simulink model "test_final_sift"  (R2015a)
settings: Solver=ode45  StartTime=0.0  StopTime=10.0  RelTol=1e-3
InitFcn:
  | %% DSPBuilder Start
  | alt_dspbuilder_update_model(bdroot)
  | %% DSPBuilder End
libraries: allblocks_alteradspbuilder2 x2309
(part 2 of 27)

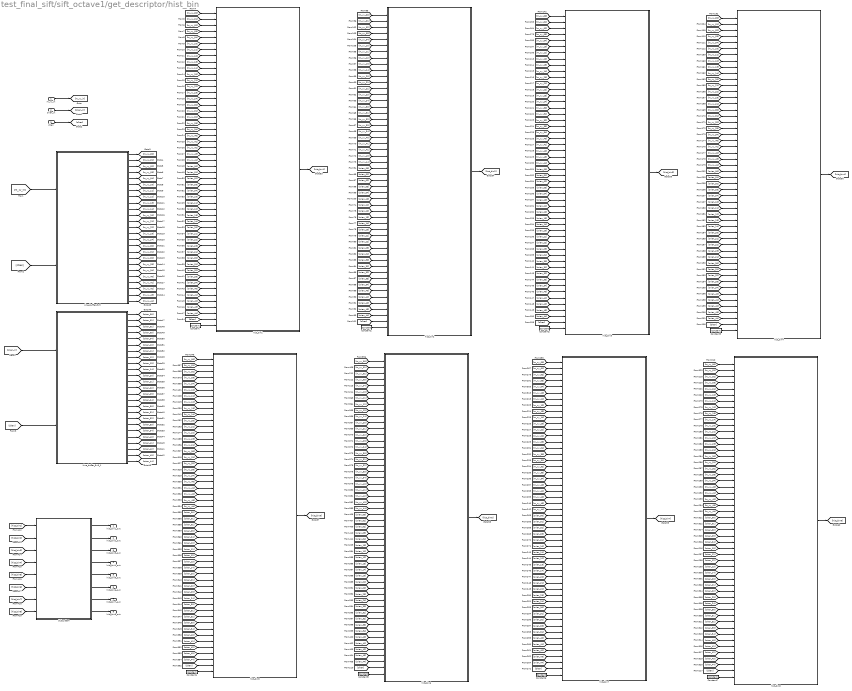
== system test_final_sift/sift_octave1/get_descriptor/hist_bin ==
  m_xy_In : Inport
  orien_In : Inport  Port=2
  clken : Inport  Port=3
  Constant : allblocks_alteradspbuilder2/Constant  mask_cst=1  BusType=Unsigned Integer  bwl=8  bwr=0  roundMode=Truncate  satMode=Wrap  SpecifyClock=off  allowFloatingPointOverride=on  logOutputs=off  logFile=C:\Users\ASUS\Desktop\sift_fpga\Octave_2\tb_test_final_sift\test%5Ffinal%5Fsift_sift%5Foctave1_get%5Fdescriptor_hist%5Fbin_Constant.fixedpointlog
  Constant1 : allblocks_alteradspbuilder2/Constant  mask_cst=2  BusType=Unsigned Integer  bwl=8  bwr=0  roundMode=Truncate  satMode=Wrap  SpecifyClock=off  allowFloatingPointOverride=on  logOutputs=off  logFile=C:\Users\ASUS\Desktop\sift_fpga\Octave_2\tb_test_final_sift\test%5Ffinal%5Fsift_sift%5Foctave1_get%5Fdescriptor_hist%5Fbin_Constant1.fixedpointlog
  Constant2 : allblocks_alteradspbuilder2/Constant  mask_cst=3  BusType=Unsigned Integer  bwl=8  bwr=0  roundMode=Truncate  satMode=Wrap  SpecifyClock=off  allowFloatingPointOverride=on  logOutputs=off  logFile=C:\Users\ASUS\Desktop\sift_fpga\Octave_2\tb_test_final_sift\test%5Ffinal%5Fsift_sift%5Foctave1_get%5Fdescriptor_hist%5Fbin_Constant2.fixedpointlog
  Constant3 : allblocks_alteradspbuilder2/Constant  mask_cst=4  BusType=Unsigned Integer  bwl=8  bwr=0  roundMode=Truncate  satMode=Wrap  SpecifyClock=off  allowFloatingPointOverride=on  logOutputs=off  logFile=C:\Users\ASUS\Desktop\sift_fpga\Octave_2\tb_test_final_sift\test%5Ffinal%5Fsift_sift%5Foctave1_get%5Fdescriptor_hist%5Fbin_Constant3.fixedpointlog
  Constant4 : allblocks_alteradspbuilder2/Constant  mask_cst=5  BusType=Unsigned Integer  bwl=8  bwr=0  roundMode=Truncate  satMode=Wrap  SpecifyClock=off  allowFloatingPointOverride=on  logOutputs=off  logFile=C:\Users\ASUS\Desktop\sift_fpga\Octave_2\tb_test_final_sift\test%5Ffinal%5Fsift_sift%5Foctave1_get%5Fdescriptor_hist%5Fbin_Constant4.fixedpointlog
  Constant5 : allblocks_alteradspbuilder2/Constant  mask_cst=6  BusType=Unsigned Integer  bwl=8  bwr=0  roundMode=Truncate  satMode=Wrap  SpecifyClock=off  allowFloatingPointOverride=on  logOutputs=off  logFile=C:\Users\ASUS\Desktop\sift_fpga\Octave_2\tb_test_final_sift\test%5Ffinal%5Fsift_sift%5Foctave1_get%5Fdescriptor_hist%5Fbin_Constant5.fixedpointlog
  Constant6 : allblocks_alteradspbuilder2/Constant  mask_cst=7  BusType=Unsigned Integer  bwl=8  bwr=0  roundMode=Truncate  satMode=Wrap  SpecifyClock=off  allowFloatingPointOverride=on  logOutputs=off  logFile=C:\Users\ASUS\Desktop\sift_fpga\Octave_2\tb_test_final_sift\test%5Ffinal%5Fsift_sift%5Foctave1_get%5Fdescriptor_hist%5Fbin_Constant6.fixedpointlog
  Constant7 : allblocks_alteradspbuilder2/Constant  mask_cst=8  BusType=Unsigned Integer  bwl=8  bwr=0  roundMode=Truncate  satMode=Wrap  SpecifyClock=off  allowFloatingPointOverride=on  logOutputs=off  logFile=C:\Users\ASUS\Desktop\sift_fpga\Octave_2\tb_test_final_sift\test%5Ffinal%5Fsift_sift%5Foctave1_get%5Fdescriptor_hist%5Fbin_Constant7.fixedpointlog
  Line_buffer_5x5 : Subsystem
  Line_buffer_5x5_1 : Subsystem
  Subsystem : Subsystem
  hist_bin1 : Subsystem
  hist_bin2 : Subsystem
  hist_bin3 : Subsystem
  hist_bin4 : Subsystem
  hist_bin5 : Subsystem
  hist_bin6 : Subsystem
  hist_bin7 : Subsystem
  hist_bin8 : Subsystem
  hist_bin1_out : Outport
  hist_bin2_out : Outport  Port=2
  hist_bin3_out : Outport  Port=3
  hist_bin4_out : Outport  Port=4
  hist_bin5_out : Outport  Port=5
  hist_bin6_out : Outport  Port=6
  hist_bin7_out : Outport  Port=7
  hist_bin8_out : Outport  Port=8
  wires:
  [hist_bin7] -> Subsystem/7(hist_in_bin7)
  [m_xy_in] -> Line_buffer_5x5/1(dataIn)
  [clken] -> Line_buffer_5x5/2(clken)
  [clken] -> Line_buffer_5x5_1/2(clken)
  [orien_in] -> Line_buffer_5x5_1/1(dataIn)
  clken/1 -> [clken]
  Line_buffer_5x5_1/21(Out40) -> [orien_40]
  Line_buffer_5x5_1/19(Out33) -> [orien_33]
  Line_buffer_5x5_1/8(Out12) -> [orien_12]
  Line_buffer_5x5_1/14(Out23) -> [orien_23]
  Line_buffer_5x5_1/18(Out32) -> [orien_32]
  Line_buffer_5x5_1/20(Out34) -> [orien_34]
  Line_buffer_5x5_1/2(Out01) -> [orien_01]
  Line_buffer_5x5_1/7(Out11) -> [orien_11]
  Line_buffer_5x5_1/11(Out20) -> [orien_20]
  Line_buffer_5x5_1/13(Out22) -> [orien_22]
  Line_buffer_5x5_1/17(Out31) -> [orien_31]
  Line_buffer_5x5_1/25(Out44) -> [orien_44]
  Line_buffer_5x5_1/3(Out02) -> [orien_02]
  Line_buffer_5x5_1/5(Out04) -> [orien_04]
  Line_buffer_5x5_1/23(Out42) -> [orien_42]
  Line_buffer_5x5_1/24(Out43) -> [orien_43]
  Line_buffer_5x5_1/6(Out10) -> [orien_10]
  Line_buffer_5x5_1/1(Out00) -> [orien_00]
  Line_buffer_5x5_1/22(Out41) -> [orien_41]
  Line_buffer_5x5_1/15(Out24) -> [orien_24]
  Line_buffer_5x5_1/4(Out03) -> [orien_03]
  Line_buffer_5x5_1/9(Out13) -> [orien_13]
  Line_buffer_5x5_1/10(Out14) -> [orien_14]
  Line_buffer_5x5_1/12(Out21) -> [orien_21]
  Line_buffer_5x5_1/16(Out30) -> [orien_30]
  Line_buffer_5x5/24(Out43) -> [m_xy_43]
  Line_buffer_5x5/21(Out40) -> [m_xy_40]
  Line_buffer_5x5/23(Out42) -> [m_xy_42]
  Line_buffer_5x5/22(Out41) -> [m_xy_41]
  Line_buffer_5x5/25(Out44) -> [m_xy_44]
  Line_buffer_5x5/12(Out21) -> [m_xy_21]
  Line_buffer_5x5/15(Out24) -> [m_xy_24]
  Line_buffer_5x5/19(Out33) -> [m_xy_33]
  Line_buffer_5x5/18(Out32) -> [m_xy_32]
  Line_buffer_5x5/13(Out22) -> [m_xy_22]
  Line_buffer_5x5/11(Out20) -> [m_xy_20]
  Line_buffer_5x5/16(Out30) -> [m_xy_30]
  Line_buffer_5x5/14(Out23) -> [m_xy_23]
  Line_buffer_5x5/17(Out31) -> [m_xy_31]
  Line_buffer_5x5/20(Out34) -> [m_xy_34]
  [hist_bin1] -> Subsystem/1(hist_in_bin1)
  Line_buffer_5x5/1(Out00) -> [m_xy_00]
  [m_xy_04] -> hist_bin1/5(Mxy_In04)
  Line_buffer_5x5/2(Out01) -> [m_xy_01]
  hist_bin1/1(bin_out) -> [hist_bin1]
  [m_xy_10] -> hist_bin1/6(Mxy_In10)
  Line_buffer_5x5/9(Out13) -> [m_xy_13]
  [m_xy_13] -> hist_bin1/9(Mxy_In13)
  Line_buffer_5x5/10(Out14) -> [m_xy_14]
  Line_buffer_5x5/6(Out10) -> [m_xy_10]
  Line_buffer_5x5/7(Out11) -> [m_xy_11]
  [m_xy_11] -> hist_bin1/7(Mxy_In11)
  [m_xy_12] -> hist_bin1/8(Mxy_In12)
  Line_buffer_5x5/8(Out12) -> [m_xy_12]
  [m_xy_14] -> hist_bin1/10(Mxy_In14)
  [m_xy_22] -> hist_bin1/13(Mxy_In22)
  [m_xy_40] -> hist_bin1/21(Mxy_In40)
  [m_xy_43] -> hist_bin1/24(Mxy_In43)
  [m_xy_42] -> hist_bin1/23(Mxy_In42)
  [m_xy_44] -> hist_bin1/25(Mxy_In44)
  [m_xy_24] -> hist_bin1/15(Mxy_In24)
  [m_xy_21] -> hist_bin1/12(Mxy_In21)
  [m_xy_20] -> hist_bin1/11(Mxy_In20)
  [m_xy_23] -> hist_bin1/14(Mxy_In23)
  [m_xy_41] -> hist_bin1/22(Mxy_In41)
  [m_xy_01] -> hist_bin1/2(Mxy_In01)
  Line_buffer_5x5/4(Out03) -> [m_xy_03]
  Line_buffer_5x5/5(Out04) -> [m_xy_04]
  Line_buffer_5x5/3(Out02) -> [m_xy_02]
  [m_xy_31] -> hist_bin1/17(Mxy_In31)
  [m_xy_30] -> hist_bin1/16(Mxy_In30)
  [m_xy_34] -> hist_bin1/20(Mxy_In34)
  [m_xy_33] -> hist_bin1/19(Mxy_In33)
  [m_xy_32] -> hist_bin1/18(Mxy_In32)
  [m_xy_03] -> hist_bin1/4(Mxy_In03)
  [m_xy_02] -> hist_bin1/3(Mxy_In02)
  [hist_bin3] -> Subsystem/3(hist_in_bin3)
  [hist_bin4] -> Subsystem/4(hist_in_bin4)
  [orien_10] -> hist_bin1/31(Orien_In10)
  [orien_42] -> hist_bin1/48(Orien_In42)
  [orien_01] -> hist_bin1/27(Orien_In01)
  [orien_20] -> hist_bin1/36(Orien_In20)
  [orien_31] -> hist_bin1/42(Orien_In31)
  [orien_33] -> hist_bin1/44(Orien_In33)
  [orien_21] -> hist_bin1/37(Orien_In21)
  [orien_24] -> hist_bin1/40(Orien_In24)
  [orien_03] -> hist_bin1/29(Orien_In03)
  [orien_30] -> hist_bin1/41(Orien_In30)
  [orien_12] -> hist_bin1/33(Orien_In12)
  [orien_23] -> hist_bin1/39(Orien_In23)
  [orien_32] -> hist_bin1/43(Orien_In32)
  [orien_41] -> hist_bin1/47(Orien_In41)
  [orien_43] -> hist_bin1/49(Orien_In43)
  [orien_02] -> hist_bin1/28(Orien_In02)
  [orien_00] -> hist_bin1/26(Orien_In00)
  [orien_11] -> hist_bin1/32(Orien_In11)
  [orien_34] -> hist_bin1/45(Orien_In34)
  [orien_22] -> hist_bin1/38(Orien_In22)
  [orien_04] -> hist_bin1/30(Orien_In04)
  [orien_14] -> hist_bin1/35(Orien_In14)
  [orien_44] -> hist_bin1/50(Orien_In44)
  [orien_13] -> hist_bin1/34(Orien_In13)
  [orien_40] -> hist_bin1/46(Orien_In40)
  [clken] -> hist_bin1/51(clken)
  Constant/1 -> hist_bin1/52(bin_in)
  [m_xy_02] -> hist_bin2/3(Mxy_In02)
  [m_xy_04] -> hist_bin2/5(Mxy_In04)
  [m_xy_10] -> hist_bin2/6(Mxy_In10)
  [m_xy_23] -> hist_bin2/14(Mxy_In23)
  [m_xy_31] -> hist_bin2/17(Mxy_In31)
  [m_xy_30] -> hist_bin2/16(Mxy_In30)
  [m_xy_12] -> hist_bin2/8(Mxy_In12)
  [m_xy_32] -> hist_bin2/18(Mxy_In32)
  [m_xy_13] -> hist_bin2/9(Mxy_In13)
  [m_xy_33] -> hist_bin2/19(Mxy_In33)
  [m_xy_41] -> hist_bin2/22(Mxy_In41)
  [m_xy_01] -> hist_bin2/2(Mxy_In01)
  [m_xy_14] -> hist_bin2/10(Mxy_In14)
  [m_xy_40] -> hist_bin2/21(Mxy_In40)
  [m_xy_43] -> hist_bin2/24(Mxy_In43)
  [m_xy_20] -> hist_bin2/11(Mxy_In20)
  [m_xy_22] -> hist_bin2/13(Mxy_In22)
  [m_xy_24] -> hist_bin2/15(Mxy_In24)
  [m_xy_34] -> hist_bin2/20(Mxy_In34)
  [m_xy_03] -> hist_bin2/4(Mxy_In03)
  [m_xy_00] -> hist_bin2/1(Mxy_In00)
  [m_xy_11] -> hist_bin2/7(Mxy_In11)
  [m_xy_21] -> hist_bin2/12(Mxy_In21)
  [orien_31] -> hist_bin2/42(Orien_In31)
  [orien_34] -> hist_bin2/45(Orien_In34)
  [m_xy_42] -> hist_bin2/23(Mxy_In42)
  [orien_01] -> hist_bin2/27(Orien_In01)
  [orien_00] -> hist_bin2/26(Orien_In00)
  [orien_04] -> hist_bin2/30(Orien_In04)
  [orien_13] -> hist_bin2/34(Orien_In13)
  [orien_20] -> hist_bin2/36(Orien_In20)
  [orien_24] -> hist_bin2/40(Orien_In24)
  [orien_33] -> hist_bin2/44(Orien_In33)
  [orien_32] -> hist_bin2/43(Orien_In32)
  [orien_41] -> hist_bin2/47(Orien_In41)
  [orien_11] -> hist_bin2/32(Orien_In11)
  [orien_21] -> hist_bin2/37(Orien_In21)
  [orien_14] -> hist_bin2/35(Orien_In14)
  [orien_22] -> hist_bin2/38(Orien_In22)
  [orien_23] -> hist_bin2/39(Orien_In23)
  [orien_02] -> hist_bin2/28(Orien_In02)
  [orien_10] -> hist_bin2/31(Orien_In10)
  [orien_12] -> hist_bin2/33(Orien_In12)
  [orien_30] -> hist_bin2/41(Orien_In30)
  [m_xy_44] -> hist_bin2/25(Mxy_In44)
  [orien_03] -> hist_bin2/29(Orien_In03)
  [orien_40] -> hist_bin2/46(Orien_In40)
  [clken] -> hist_bin2/51(clken)
  hist_bin2/1(bin_out) -> [hist_bin2]
  [orien_42] -> hist_bin2/48(Orien_In42)
  [orien_44] -> hist_bin2/50(Orien_In44)
  [orien_43] -> hist_bin2/49(Orien_In43)
  Constant1/1 -> hist_bin2/52(bin_in)
  [m_xy_00] -> hist_bin1/1(Mxy_In00)
  Subsystem/4(bin4_out) -> hist_bin4_out/1
  Subsystem/3(bin3_out) -> hist_bin3_out/1
  [hist_bin8] -> Subsystem/8(hist_in_bin8)
  [hist_bin6] -> Subsystem/6(hist_in_bin6)
  [hist_bin5] -> Subsystem/5(hist_in_bin5)
  Subsystem/2(bin2_out) -> hist_bin2_out/1
  orien_In/1 -> [orien_in]
  m_xy_In/1 -> [m_xy_in]
  Subsystem/5(bin5_out) -> hist_bin5_out/1
  Subsystem/6(bin6_out) -> hist_bin6_out/1
  Subsystem/7(bin7_out) -> hist_bin7_out/1
  Subsystem/8(bin8_out) -> hist_bin8_out/1
  [hist_bin2] -> Subsystem/2(hist_in_bin2)
  [m_xy_04] -> hist_bin3/5(Mxy_In04)
  hist_bin3/1(bin_out) -> [hist_bin3]
  [m_xy_10] -> hist_bin3/6(Mxy_In10)
  [m_xy_13] -> hist_bin3/9(Mxy_In13)
  [m_xy_11] -> hist_bin3/7(Mxy_In11)
  [m_xy_12] -> hist_bin3/8(Mxy_In12)
  [m_xy_14] -> hist_bin3/10(Mxy_In14)
  [m_xy_22] -> hist_bin3/13(Mxy_In22)
  [m_xy_40] -> hist_bin3/21(Mxy_In40)
  [m_xy_43] -> hist_bin3/24(Mxy_In43)
  [m_xy_42] -> hist_bin3/23(Mxy_In42)
  [m_xy_44] -> hist_bin3/25(Mxy_In44)
  [m_xy_24] -> hist_bin3/15(Mxy_In24)
  [m_xy_21] -> hist_bin3/12(Mxy_In21)
  [m_xy_20] -> hist_bin3/11(Mxy_In20)
  [m_xy_23] -> hist_bin3/14(Mxy_In23)
  [m_xy_41] -> hist_bin3/22(Mxy_In41)
  [m_xy_01] -> hist_bin3/2(Mxy_In01)
  [m_xy_31] -> hist_bin3/17(Mxy_In31)
  [m_xy_30] -> hist_bin3/16(Mxy_In30)
  [m_xy_34] -> hist_bin3/20(Mxy_In34)
  [m_xy_33] -> hist_bin3/19(Mxy_In33)
  [m_xy_32] -> hist_bin3/18(Mxy_In32)
  [m_xy_03] -> hist_bin3/4(Mxy_In03)
  [m_xy_02] -> hist_bin3/3(Mxy_In02)
  [orien_10] -> hist_bin3/31(Orien_In10)
  [orien_42] -> hist_bin3/48(Orien_In42)
  [orien_01] -> hist_bin3/27(Orien_In01)
  [orien_20] -> hist_bin3/36(Orien_In20)
  [orien_31] -> hist_bin3/42(Orien_In31)
  [orien_33] -> hist_bin3/44(Orien_In33)
  [orien_21] -> hist_bin3/37(Orien_In21)
  [orien_24] -> hist_bin3/40(Orien_In24)
  [orien_03] -> hist_bin3/29(Orien_In03)
  [orien_30] -> hist_bin3/41(Orien_In30)
  [orien_12] -> hist_bin3/33(Orien_In12)
  [orien_23] -> hist_bin3/39(Orien_In23)
  [orien_32] -> hist_bin3/43(Orien_In32)
  [orien_41] -> hist_bin3/47(Orien_In41)
  [orien_43] -> hist_bin3/49(Orien_In43)
  [orien_02] -> hist_bin3/28(Orien_In02)
  [orien_00] -> hist_bin3/26(Orien_In00)
  [orien_11] -> hist_bin3/32(Orien_In11)
  [orien_34] -> hist_bin3/45(Orien_In34)
  [orien_22] -> hist_bin3/38(Orien_In22)
  [orien_04] -> hist_bin3/30(Orien_In04)
  [orien_14] -> hist_bin3/35(Orien_In14)
  [orien_44] -> hist_bin3/50(Orien_In44)
  [orien_13] -> hist_bin3/34(Orien_In13)
  [orien_40] -> hist_bin3/46(Orien_In40)
  [clken] -> hist_bin3/51(clken)
  Constant2/1 -> hist_bin3/52(bin_in)
  [m_xy_02] -> hist_bin4/3(Mxy_In02)
  [m_xy_04] -> hist_bin4/5(Mxy_In04)
  [m_xy_10] -> hist_bin4/6(Mxy_In10)
  [m_xy_23] -> hist_bin4/14(Mxy_In23)
  [m_xy_31] -> hist_bin4/17(Mxy_In31)
  [m_xy_30] -> hist_bin4/16(Mxy_In30)
  [m_xy_12] -> hist_bin4/8(Mxy_In12)
  [m_xy_32] -> hist_bin4/18(Mxy_In32)
  [m_xy_13] -> hist_bin4/9(Mxy_In13)
  [m_xy_33] -> hist_bin4/19(Mxy_In33)
  [m_xy_41] -> hist_bin4/22(Mxy_In41)
  [m_xy_01] -> hist_bin4/2(Mxy_In01)
  [m_xy_14] -> hist_bin4/10(Mxy_In14)
  [m_xy_40] -> hist_bin4/21(Mxy_In40)
  [m_xy_43] -> hist_bin4/24(Mxy_In43)
  [m_xy_20] -> hist_bin4/11(Mxy_In20)
  [m_xy_22] -> hist_bin4/13(Mxy_In22)
  [m_xy_24] -> hist_bin4/15(Mxy_In24)
  [m_xy_34] -> hist_bin4/20(Mxy_In34)
  [m_xy_03] -> hist_bin4/4(Mxy_In03)
  [m_xy_00] -> hist_bin4/1(Mxy_In00)
  [m_xy_11] -> hist_bin4/7(Mxy_In11)
  [m_xy_21] -> hist_bin4/12(Mxy_In21)
  [orien_31] -> hist_bin4/42(Orien_In31)
  [orien_34] -> hist_bin4/45(Orien_In34)
  [m_xy_42] -> hist_bin4/23(Mxy_In42)
  [orien_01] -> hist_bin4/27(Orien_In01)
  [orien_00] -> hist_bin4/26(Orien_In00)
  [orien_04] -> hist_bin4/30(Orien_In04)
  [orien_13] -> hist_bin4/34(Orien_In13)
  [orien_20] -> hist_bin4/36(Orien_In20)
  [orien_24] -> hist_bin4/40(Orien_In24)
  [orien_33] -> hist_bin4/44(Orien_In33)
  [orien_32] -> hist_bin4/43(Orien_In32)
  [orien_41] -> hist_bin4/47(Orien_In41)
  [orien_11] -> hist_bin4/32(Orien_In11)
  [orien_21] -> hist_bin4/37(Orien_In21)
  [orien_14] -> hist_bin4/35(Orien_In14)
  [orien_22] -> hist_bin4/38(Orien_In22)
  [orien_23] -> hist_bin4/39(Orien_In23)
  [orien_02] -> hist_bin4/28(Orien_In02)
  [orien_10] -> hist_bin4/31(Orien_In10)
  [orien_12] -> hist_bin4/33(Orien_In12)
  [orien_30] -> hist_bin4/41(Orien_In30)
  [m_xy_44] -> hist_bin4/25(Mxy_In44)
  [orien_03] -> hist_bin4/29(Orien_In03)
  [orien_40] -> hist_bin4/46(Orien_In40)
  [clken] -> hist_bin4/51(clken)
  hist_bin4/1(bin_out) -> [hist_bin4]
  [orien_42] -> hist_bin4/48(Orien_In42)
  [orien_44] -> hist_bin4/50(Orien_In44)
  [orien_43] -> hist_bin4/49(Orien_In43)
  Constant3/1 -> hist_bin4/52(bin_in)
  [m_xy_00] -> hist_bin3/1(Mxy_In00)
  [m_xy_04] -> hist_bin5/5(Mxy_In04)
  hist_bin5/1(bin_out) -> [hist_bin5]
  [m_xy_10] -> hist_bin5/6(Mxy_In10)
  [m_xy_13] -> hist_bin5/9(Mxy_In13)
  [m_xy_11] -> hist_bin5/7(Mxy_In11)
  [m_xy_12] -> hist_bin5/8(Mxy_In12)
  [m_xy_14] -> hist_bin5/10(Mxy_In14)
  [m_xy_22] -> hist_bin5/13(Mxy_In22)
  [m_xy_40] -> hist_bin5/21(Mxy_In40)
  [m_xy_43] -> hist_bin5/24(Mxy_In43)
  [m_xy_42] -> hist_bin5/23(Mxy_In42)
  [m_xy_44] -> hist_bin5/25(Mxy_In44)
  [m_xy_24] -> hist_bin5/15(Mxy_In24)
  [m_xy_21] -> hist_bin5/12(Mxy_In21)
  [m_xy_20] -> hist_bin5/11(Mxy_In20)
  [m_xy_23] -> hist_bin5/14(Mxy_In23)
  [m_xy_41] -> hist_bin5/22(Mxy_In41)
  [m_xy_01] -> hist_bin5/2(Mxy_In01)
  [m_xy_31] -> hist_bin5/17(Mxy_In31)
  [m_xy_30] -> hist_bin5/16(Mxy_In30)
  [m_xy_34] -> hist_bin5/20(Mxy_In34)
  [m_xy_33] -> hist_bin5/19(Mxy_In33)
  [m_xy_32] -> hist_bin5/18(Mxy_In32)
  [m_xy_03] -> hist_bin5/4(Mxy_In03)
  [m_xy_02] -> hist_bin5/3(Mxy_In02)
  [orien_10] -> hist_bin5/31(Orien_In10)
  [orien_42] -> hist_bin5/48(Orien_In42)
  [orien_01] -> hist_bin5/27(Orien_In01)
  [orien_20] -> hist_bin5/36(Orien_In20)
  [orien_31] -> hist_bin5/42(Orien_In31)
  [orien_33] -> hist_bin5/44(Orien_In33)
  [orien_21] -> hist_bin5/37(Orien_In21)
  [orien_24] -> hist_bin5/40(Orien_In24)
  [orien_03] -> hist_bin5/29(Orien_In03)
  [orien_30] -> hist_bin5/41(Orien_In30)
  [orien_12] -> hist_bin5/33(Orien_In12)
  [orien_23] -> hist_bin5/39(Orien_In23)
  [orien_32] -> hist_bin5/43(Orien_In32)
  [orien_41] -> hist_bin5/47(Orien_In41)
  [orien_43] -> hist_bin5/49(Orien_In43)
  [orien_02] -> hist_bin5/28(Orien_In02)
  [orien_00] -> hist_bin5/26(Orien_In00)
  [orien_11] -> hist_bin5/32(Orien_In11)
  [orien_34] -> hist_bin5/45(Orien_In34)
  [orien_22] -> hist_bin5/38(Orien_In22)
  [orien_04] -> hist_bin5/30(Orien_In04)
  [orien_14] -> hist_bin5/35(Orien_In14)
  [orien_44] -> hist_bin5/50(Orien_In44)
  [orien_13] -> hist_bin5/34(Orien_In13)
  [orien_40] -> hist_bin5/46(Orien_In40)
  [clken] -> hist_bin5/51(clken)
  Constant4/1 -> hist_bin5/52(bin_in)
  [m_xy_02] -> hist_bin6/3(Mxy_In02)
  [m_xy_04] -> hist_bin6/5(Mxy_In04)
  [m_xy_10] -> hist_bin6/6(Mxy_In10)
  [m_xy_23] -> hist_bin6/14(Mxy_In23)
  [m_xy_31] -> hist_bin6/17(Mxy_In31)
  [m_xy_30] -> hist_bin6/16(Mxy_In30)
  [m_xy_12] -> hist_bin6/8(Mxy_In12)
  [m_xy_32] -> hist_bin6/18(Mxy_In32)
  [m_xy_13] -> hist_bin6/9(Mxy_In13)
  [m_xy_33] -> hist_bin6/19(Mxy_In33)
  [m_xy_41] -> hist_bin6/22(Mxy_In41)
  [m_xy_01] -> hist_bin6/2(Mxy_In01)
  [m_xy_14] -> hist_bin6/10(Mxy_In14)
  [m_xy_40] -> hist_bin6/21(Mxy_In40)
  [m_xy_43] -> hist_bin6/24(Mxy_In43)
  [m_xy_20] -> hist_bin6/11(Mxy_In20)
  [m_xy_22] -> hist_bin6/13(Mxy_In22)
  [m_xy_24] -> hist_bin6/15(Mxy_In24)
  [m_xy_34] -> hist_bin6/20(Mxy_In34)
  [m_xy_03] -> hist_bin6/4(Mxy_In03)
  [m_xy_00] -> hist_bin6/1(Mxy_In00)
  [m_xy_11] -> hist_bin6/7(Mxy_In11)
  [m_xy_21] -> hist_bin6/12(Mxy_In21)
  [orien_31] -> hist_bin6/42(Orien_In31)
  [orien_34] -> hist_bin6/45(Orien_In34)
  [m_xy_42] -> hist_bin6/23(Mxy_In42)
  [orien_01] -> hist_bin6/27(Orien_In01)
  [orien_00] -> hist_bin6/26(Orien_In00)
  [orien_04] -> hist_bin6/30(Orien_In04)
  [orien_13] -> hist_bin6/34(Orien_In13)
  [orien_20] -> hist_bin6/36(Orien_In20)
  [orien_24] -> hist_bin6/40(Orien_In24)
  [orien_33] -> hist_bin6/44(Orien_In33)
  [orien_32] -> hist_bin6/43(Orien_In32)
  [orien_41] -> hist_bin6/47(Orien_In41)
  [orien_11] -> hist_bin6/32(Orien_In11)
  [orien_21] -> hist_bin6/37(Orien_In21)
  [orien_14] -> hist_bin6/35(Orien_In14)
  [orien_22] -> hist_bin6/38(Orien_In22)
  [orien_23] -> hist_bin6/39(Orien_In23)
  [orien_02] -> hist_bin6/28(Orien_In02)
  [orien_10] -> hist_bin6/31(Orien_In10)
  [orien_12] -> hist_bin6/33(Orien_In12)
  [orien_30] -> hist_bin6/41(Orien_In30)
  [m_xy_44] -> hist_bin6/25(Mxy_In44)
  [orien_03] -> hist_bin6/29(Orien_In03)
  [orien_40] -> hist_bin6/46(Orien_In40)
  [clken] -> hist_bin6/51(clken)
  hist_bin6/1(bin_out) -> [hist_bin6]
  [orien_42] -> hist_bin6/48(Orien_In42)
  [orien_44] -> hist_bin6/50(Orien_In44)
  [orien_43] -> hist_bin6/49(Orien_In43)
  Constant5/1 -> hist_bin6/52(bin_in)
  [m_xy_00] -> hist_bin5/1(Mxy_In00)
  [m_xy_04] -> hist_bin7/5(Mxy_In04)
  hist_bin7/1(bin_out) -> [hist_bin7]
  [m_xy_10] -> hist_bin7/6(Mxy_In10)
  [m_xy_13] -> hist_bin7/9(Mxy_In13)
  [m_xy_11] -> hist_bin7/7(Mxy_In11)
  [m_xy_12] -> hist_bin7/8(Mxy_In12)
  [m_xy_14] -> hist_bin7/10(Mxy_In14)
  [m_xy_22] -> hist_bin7/13(Mxy_In22)
  [m_xy_40] -> hist_bin7/21(Mxy_In40)
  [m_xy_43] -> hist_bin7/24(Mxy_In43)
  [m_xy_42] -> hist_bin7/23(Mxy_In42)
  [m_xy_44] -> hist_bin7/25(Mxy_In44)
  [m_xy_24] -> hist_bin7/15(Mxy_In24)
  [m_xy_21] -> hist_bin7/12(Mxy_In21)
  [m_xy_20] -> hist_bin7/11(Mxy_In20)
  [m_xy_23] -> hist_bin7/14(Mxy_In23)
  [m_xy_41] -> hist_bin7/22(Mxy_In41)
  [m_xy_01] -> hist_bin7/2(Mxy_In01)
  [m_xy_31] -> hist_bin7/17(Mxy_In31)
  [m_xy_30] -> hist_bin7/16(Mxy_In30)
  [m_xy_34] -> hist_bin7/20(Mxy_In34)
  [m_xy_33] -> hist_bin7/19(Mxy_In33)
  [m_xy_32] -> hist_bin7/18(Mxy_In32)
  [m_xy_03] -> hist_bin7/4(Mxy_In03)
  [m_xy_02] -> hist_bin7/3(Mxy_In02)
  [orien_10] -> hist_bin7/31(Orien_In10)
  [orien_42] -> hist_bin7/48(Orien_In42)
  [orien_01] -> hist_bin7/27(Orien_In01)
  [orien_20] -> hist_bin7/36(Orien_In20)
  [orien_31] -> hist_bin7/42(Orien_In31)
  [orien_33] -> hist_bin7/44(Orien_In33)
  [orien_21] -> hist_bin7/37(Orien_In21)
  [orien_24] -> hist_bin7/40(Orien_In24)
  [orien_03] -> hist_bin7/29(Orien_In03)
  [orien_30] -> hist_bin7/41(Orien_In30)
  [orien_12] -> hist_bin7/33(Orien_In12)
  [orien_23] -> hist_bin7/39(Orien_In23)
  [orien_32] -> hist_bin7/43(Orien_In32)
  [orien_41] -> hist_bin7/47(Orien_In41)
  [orien_43] -> hist_bin7/49(Orien_In43)
  [orien_02] -> hist_bin7/28(Orien_In02)
  [orien_00] -> hist_bin7/26(Orien_In00)
  [orien_11] -> hist_bin7/32(Orien_In11)
  [orien_34] -> hist_bin7/45(Orien_In34)
  [orien_22] -> hist_bin7/38(Orien_In22)
  [orien_04] -> hist_bin7/30(Orien_In04)
  [orien_14] -> hist_bin7/35(Orien_In14)
  [orien_44] -> hist_bin7/50(Orien_In44)
  [orien_13] -> hist_bin7/34(Orien_In13)
  [orien_40] -> hist_bin7/46(Orien_In40)
  [clken] -> hist_bin7/51(clken)
  Constant6/1 -> hist_bin7/52(bin_in)
  [m_xy_02] -> hist_bin8/3(Mxy_In02)
  [m_xy_04] -> hist_bin8/5(Mxy_In04)
  [m_xy_10] -> hist_bin8/6(Mxy_In10)
  [m_xy_23] -> hist_bin8/14(Mxy_In23)
  [m_xy_31] -> hist_bin8/17(Mxy_In31)
  [m_xy_30] -> hist_bin8/16(Mxy_In30)
  [m_xy_12] -> hist_bin8/8(Mxy_In12)
  [m_xy_32] -> hist_bin8/18(Mxy_In32)
  [m_xy_13] -> hist_bin8/9(Mxy_In13)
  [m_xy_33] -> hist_bin8/19(Mxy_In33)
  [m_xy_41] -> hist_bin8/22(Mxy_In41)
  [m_xy_01] -> hist_bin8/2(Mxy_In01)
  [m_xy_14] -> hist_bin8/10(Mxy_In14)
  [m_xy_40] -> hist_bin8/21(Mxy_In40)
  [m_xy_43] -> hist_bin8/24(Mxy_In43)
  [m_xy_20] -> hist_bin8/11(Mxy_In20)
  [m_xy_22] -> hist_bin8/13(Mxy_In22)
  [m_xy_24] -> hist_bin8/15(Mxy_In24)
  [m_xy_34] -> hist_bin8/20(Mxy_In34)
  [m_xy_03] -> hist_bin8/4(Mxy_In03)
  [m_xy_00] -> hist_bin8/1(Mxy_In00)
  [m_xy_11] -> hist_bin8/7(Mxy_In11)
  [m_xy_21] -> hist_bin8/12(Mxy_In21)
  [orien_31] -> hist_bin8/42(Orien_In31)
  [orien_34] -> hist_bin8/45(Orien_In34)
  [m_xy_42] -> hist_bin8/23(Mxy_In42)
  [orien_01] -> hist_bin8/27(Orien_In01)
  [orien_00] -> hist_bin8/26(Orien_In00)
  [orien_04] -> hist_bin8/30(Orien_In04)
  [orien_13] -> hist_bin8/34(Orien_In13)
  [orien_20] -> hist_bin8/36(Orien_In20)
  [orien_24] -> hist_bin8/40(Orien_In24)
  [orien_33] -> hist_bin8/44(Orien_In33)
  [orien_32] -> hist_bin8/43(Orien_In32)
  [orien_41] -> hist_bin8/47(Orien_In41)
  [orien_11] -> hist_bin8/32(Orien_In11)
  [orien_21] -> hist_bin8/37(Orien_In21)
  [orien_14] -> hist_bin8/35(Orien_In14)
  [orien_22] -> hist_bin8/38(Orien_In22)
  [orien_23] -> hist_bin8/39(Orien_In23)
  [orien_02] -> hist_bin8/28(Orien_In02)
  [orien_10] -> hist_bin8/31(Orien_In10)
  [orien_12] -> hist_bin8/33(Orien_In12)
  [orien_30] -> hist_bin8/41(Orien_In30)
  [m_xy_44] -> hist_bin8/25(Mxy_In44)
  [orien_03] -> hist_bin8/29(Orien_In03)
  [orien_40] -> hist_bin8/46(Orien_In40)
  [clken] -> hist_bin8/51(clken)
  hist_bin8/1(bin_out) -> [hist_bin8]
  [orien_42] -> hist_bin8/48(Orien_In42)
  [orien_44] -> hist_bin8/50(Orien_In44)
  [orien_43] -> hist_bin8/49(Orien_In43)
  Constant7/1 -> hist_bin8/52(bin_in)
  [m_xy_00] -> hist_bin7/1(Mxy_In00)
  Subsystem/1(bin1_out) -> hist_bin1_out/1

== system test_final_sift/sift_octave1/get_descriptor/scale_space ==
  data_in : Inport
  valid_in : Inport  Port=2
  Gaussian_scale1 : Subsystem
  Gaussian_scale2 : Subsystem
  Gaussian_scale3 : Subsystem
  Gaussian_scale4 : Subsystem
  scale4 : Outport
  scale3 : Outport  Port=2
  scale2 : Outport  Port=3
  scale1 : Outport  Port=4
  wires:
  data_in/1 -> [pixel_in]
  valid_in/1 -> [valid_in]
  [pixel_in] -> Gaussian_scale3/1(pixel_in)
  [pixel_in] -> Gaussian_scale4/1(pixel_in)
  [valid_in] -> Gaussian_scale3/2(valid_in)
  [pixel_in] -> Gaussian_scale1/1(pixel_in)
  [valid_in] -> Gaussian_scale1/2(valid_in)
  [valid_in] -> Gaussian_scale4/2(valid_in)
  [pixel_in] -> Gaussian_scale2/1(pixel_in)
  [valid_in] -> Gaussian_scale2/2(valid_in)
  Gaussian_scale3/1(pixel_out) -> [pixel_scale3]
  [pixel_scale3] -> scale3/1
  [pixel_scale2] -> scale2/1
  Gaussian_scale4/1(pixel_out) -> [pixel_scale4]
  [pixel_scale4] -> scale4/1
  Gaussian_scale1/1(pixel_out) -> [pixel_scale1]
  Gaussian_scale2/1(pixel_out) -> [pixel_scale2]
  [pixel_scale1] -> scale1/1

== system test_final_sift/sift_octave1/matching/Ram ==
  descriptor : Inport
  control_write : Inport  Port=2
  eof : Inport  Port=3
  add_read_first : Inport  Port=4
  add_read_second : Inport  Port=5
  clken : Inport  Port=6
  ena_match : Inport  Port=7
  Logical Bit Operator : allblocks_alteradspbuilder2/Logical Bit Operator  LogicalOperator=AND  user_inputs=2  pipeline_display=0
  Logical Bit Operator1 : allblocks_alteradspbuilder2/Logical Bit Operator  LogicalOperator=NOT  user_inputs=2  pipeline_display=0
  Logical Bit Operator2 : allblocks_alteradspbuilder2/Logical Bit Operator  LogicalOperator=AND  user_inputs=2  pipeline_display=0
  Logical Bit Operator3 : allblocks_alteradspbuilder2/Logical Bit Operator  LogicalOperator=NOT  user_inputs=2  pipeline_display=0
  picture_first : Subsystem
  picture_second : Subsystem
  ram_descriptor_first : allblocks_alteradspbuilder2/Dual-Port RAM  numwords=1000  BusType=Signed Integer  bwl=1172  bwr=0  memory_type=AUTO  ram_type=DualRAM  dont_care=on  initialization=Blank  init_file=input.hex  init_array=[0:1:15]  register_outputs=on  use_ena=off  ClockPhase=1  allowFloatingPointOverride=on  logOutputs=off  logFile=C:\Users\ASUS\Desktop\sift_fpga\Octave_2\tb_test_final_sift\test%5Ffinal%5Fsift_sift%5Foctave1_matching_Ram_ram%5Fdescriptor%5Ffirst.fixedpointlog  pipeline_display=2
  ram_descriptor_second : allblocks_alteradspbuilder2/Dual-Port RAM  numwords=1000  BusType=Signed Integer  bwl=1172  bwr=0  memory_type=AUTO  ram_type=DualRAM  dont_care=on  initialization=Blank  init_file=input.hex  init_array=[0:1:15]  register_outputs=on  use_ena=off  ClockPhase=1  allowFloatingPointOverride=on  logOutputs=off  logFile=C:\Users\ASUS\Desktop\sift_fpga\Octave_2\tb_test_final_sift\test%5Ffinal%5Fsift_sift%5Foctave1_matching_Ram_ram%5Fdescriptor%5Fsecond.fixedpointlog  pipeline_display=2
  descriptor_first : Outport
  descriptor_second : Outport  Port=2
  wires:
  [descriptor] -> picture_first/1(descriptor)
  picture_first/2(add_write) -> ram_descriptor_first/3
  picture_first/1(data) -> ram_descriptor_first/1
  picture_first/3(ena_write) -> Logical Bit Operator/1
  [eof] -> picture_second/2(eof)
  [add_read_first] -> ram_descriptor_first/2
  ram_descriptor_first/1 -> descriptor_first/1
  ram_descriptor_second/1 -> descriptor_second/1
  [add_read_second] -> ram_descriptor_second/2
  [eof] -> picture_first/2(eof)
  picture_second/1(data) -> ram_descriptor_second/1
  picture_second/2(add_write) -> ram_descriptor_second/3
  eof/1 -> [eof]
  control_write/1 -> [allow]
  [allow] -> picture_first/4(allow)
  descriptor/1 -> [descriptor]
  add_read_first/1 -> [add_read_first]
  add_read_second/1 -> [add_read_second]
  clken/1 -> [clken]
  [clken] -> picture_first/3(clken)
  [clken] -> picture_second/3(clken)
  [descriptor] -> picture_second/1(descriptor)
  [allow] -> picture_second/4(allow)
  ena_match/1 -> [ena_match]
  Logical Bit Operator/1 -> ram_descriptor_first/4
  Logical Bit Operator1/1 -> Logical Bit Operator/2
  [ena_match] -> Logical Bit Operator1/1
  picture_second/3(ena_write) -> Logical Bit Operator2/1
  Logical Bit Operator2/1 -> ram_descriptor_second/4
  Logical Bit Operator3/1 -> Logical Bit Operator2/2
  [ena_match] -> Logical Bit Operator3/1

== system test_final_sift/sift_octave1/matching/Ram_location_match ==
  match : Inport
  location : Inport  Port=2
  clken : Inport  Port=3
  sclr : Inport  Port=4
  add_read_location : Inport  Port=5
  ctr_draw_match : Inport  Port=6
  Constant : allblocks_alteradspbuilder2/Constant  mask_cst=1998  BusType=Unsigned Integer  bwl=20  bwr=0  roundMode=Truncate  satMode=Wrap  SpecifyClock=off  allowFloatingPointOverride=on  logOutputs=off  logFile=C:\Users\ASUS\Desktop\sift_fpga\Octave_2\tb_test_final_sift\test%5Ffinal%5Fsift_sift%5Foctave1_matching_Ram%5Flocation%5Fmatch_Constant.fixedpointlog
  Constant1 : allblocks_alteradspbuilder2/Constant  mask_cst=1  BusType=Unsigned Integer  bwl=20  bwr=0  roundMode=Truncate  satMode=Wrap  SpecifyClock=off  allowFloatingPointOverride=on  logOutputs=off  logFile=C:\Users\ASUS\Desktop\sift_fpga\Octave_2\tb_test_final_sift\test%5Ffinal%5Fsift_sift%5Foctave1_matching_Ram%5Flocation%5Fmatch_Constant1.fixedpointlog
  Counter : allblocks_alteradspbuilder2/Counter  BusType=Unsigned Integer  bwl=10  bwr=0  use_modulo=on  modulo=1000  SpecifyClock=off  direction=Increment  use_sload=off  use_sset=off  svalue=1  use_clk_ena=off  use_ena=on  use_sclr=on  pipeline_display=1
  Dual-Port RAM : allblocks_alteradspbuilder2/Dual-Port RAM  numwords=1000  BusType=Unsigned Integer  bwl=20  bwr=0  memory_type=M9K  ram_type=DualRAM  dont_care=on  initialization=Blank  init_file=input.hex  init_array=[0:1:15]  register_outputs=on  use_ena=off  ClockPhase=1  allowFloatingPointOverride=on  logOutputs=off  logFile=C:\Users\ASUS\Desktop\sift_fpga\Octave_2\tb_test_final_sift\test%5Ffinal%5Fsift_sift%5Foctave1_matching_Ram%5Flocation%5Fmatch_Dual-Port+RAM.fixedpointlog  pipeline_display=2
  Logical Bit Operator{,1..2,4,6} (5 alike) : allblocks_alteradspbuilder2/Logical Bit Operator  LogicalOperator=AND  user_inputs=2  pipeline_display=0
  Logical Bit Operator3 : allblocks_alteradspbuilder2/Logical Bit Operator  LogicalOperator=OR  user_inputs=2  pipeline_display=0
  Logical Bit Operator5 : allblocks_alteradspbuilder2/Logical Bit Operator  LogicalOperator=OR  user_inputs=2  pipeline_display=0
  Logical Bit Operator7 : allblocks_alteradspbuilder2/Logical Bit Operator  LogicalOperator=NOT  user_inputs=2  pipeline_display=0
  Multiplexer : allblocks_alteradspbuilder2/Multiplexer  numInputs=2  pipeline=0  oneHot=off  pipeline_display=0  use_ena=off  use_aclr=off  allowFloatingPointOverride=on  logOutputs=off  logFile=C:\Users\ASUS\Desktop\sift_fpga\Octave_2\tb_test_final_sift\test%5Ffinal%5Fsift_sift%5Foctave1_matching_Ram%5Flocation%5Fmatch_Multiplexer.fixedpointlog
  Multiplexer1 : allblocks_alteradspbuilder2/Multiplexer  numInputs=2  pipeline=0  oneHot=off  pipeline_display=0  use_ena=off  use_aclr=off  allowFloatingPointOverride=on  logOutputs=off  logFile=C:\Users\ASUS\Desktop\sift_fpga\Octave_2\tb_test_final_sift\test%5Ffinal%5Fsift_sift%5Foctave1_matching_Ram%5Flocation%5Fmatch_Multiplexer1.fixedpointlog
  Parallel Adder Subtractor : allblocks_alteradspbuilder2/Parallel Adder Subtractor  number_of_inputs=2  direction=+  use_pipeline=on  pipeline_display=1  phase_selection=1  use_ena=off  use_aclr=off  allowFloatingPointOverride=on  logOutputs=off  logFile=C:\Users\ASUS\Desktop\sift_fpga\Octave_2\tb_test_final_sift\test%5Ffinal%5Fsift_sift%5Foctave1_matching_Ram%5Flocation%5Fmatch_Parallel+Adder+Subtractor.fixedpointlog
  location_out : Outport
  wires:
  match/1 -> [match]
  location/1 -> [location]
  clken/1 -> [clken]
  Logical Bit Operator/1 -> Logical Bit Operator3/1
  Counter/1 -> [addr_write]
  [match] -> Logical Bit Operator/2
  [clken] -> Logical Bit Operator/1
  Multiplexer1/1 -> Dual-Port RAM/3
  Logical Bit Operator1/1 -> Logical Bit Operator5/2
  [match] -> Logical Bit Operator1/2
  [clken] -> Logical Bit Operator1/1
  sclr/1 -> [sclr]
  [sclr] -> Logical Bit Operator2/2
  [clken] -> Logical Bit Operator2/1
  Logical Bit Operator2/1 -> Counter/2, Logical Bit Operator3/2
  add_read_location/1 -> [addr_location_r]
  [addr_location_r] -> Dual-Port RAM/2
  Dual-Port RAM/1 -> [location_out]
  [location_out] -> location_out/1
  Logical Bit Operator3/1 -> Counter/1
  [location] -> Multiplexer/2
  Constant/1 -> Multiplexer/3
  [sclr] -> Logical Bit Operator4/2
  [clken] -> Logical Bit Operator4/1
  Logical Bit Operator4/1 -> Logical Bit Operator5/1, Multiplexer1/1, Multiplexer/1
  Multiplexer/1 -> Dual-Port RAM/1
  [addr_write] -> Parallel Adder Subtractor/1
  Constant1/1 -> Parallel Adder Subtractor/2
  Parallel Adder Subtractor/1 -> [addr_final]
  Logical Bit Operator5/1 -> Logical Bit Operator6/1
  [addr_write] -> Multiplexer1/2
  [addr_final] -> Multiplexer1/3
  Logical Bit Operator6/1 -> Dual-Port RAM/4
  ctr_draw_match/1 -> [ctr_draw_match]
  [ctr_draw_match] -> Logical Bit Operator7/1
  Logical Bit Operator7/1 -> Logical Bit Operator6/2

== system test_final_sift/sift_octave1/matching/add_read_desciptor ==
  valid_in : Inport
  option_ena : Inport  Port=2
  Comparator : allblocks_alteradspbuilder2/Comparator  direction=a == b  pipeline_display=0  allowFloatingPointOverride=on  logOutputs=off  logFile=C:\Users\ASUS\Desktop\sift_fpga\Octave_2\tb_test_final_sift\test%5Ffinal%5Fsift_sift%5Foctave1_matching_add%5Fread%5Fdesciptor_Comparator.fixedpointlog
  Comparator1 : allblocks_alteradspbuilder2/Comparator  direction=a == b  pipeline_display=0  allowFloatingPointOverride=on  logOutputs=off  logFile=C:\Users\ASUS\Desktop\sift_fpga\Octave_2\tb_test_final_sift\test%5Ffinal%5Fsift_sift%5Foctave1_matching_add%5Fread%5Fdesciptor_Comparator1.fixedpointlog
  Comparator2 : allblocks_alteradspbuilder2/Comparator  direction=a == b  pipeline_display=0  allowFloatingPointOverride=on  logOutputs=off  logFile=C:\Users\ASUS\Desktop\sift_fpga\Octave_2\tb_test_final_sift\test%5Ffinal%5Fsift_sift%5Foctave1_matching_add%5Fread%5Fdesciptor_Comparator2.fixedpointlog
  Constant : allblocks_alteradspbuilder2/Constant  mask_cst=999  BusType=Unsigned Integer  bwl=10  bwr=0  roundMode=Truncate  satMode=Wrap  SpecifyClock=off  allowFloatingPointOverride=on  logOutputs=off  logFile=C:\Users\ASUS\Desktop\sift_fpga\Octave_2\tb_test_final_sift\test%5Ffinal%5Fsift_sift%5Foctave1_matching_add%5Fread%5Fdesciptor_Constant.fixedpointlog
  Constant1 : allblocks_alteradspbuilder2/Constant  mask_cst=0  BusType=Unsigned Integer  bwl=10  bwr=0  roundMode=Truncate  satMode=Wrap  SpecifyClock=off  allowFloatingPointOverride=on  logOutputs=off  logFile=C:\Users\ASUS\Desktop\sift_fpga\Octave_2\tb_test_final_sift\test%5Ffinal%5Fsift_sift%5Foctave1_matching_add%5Fread%5Fdesciptor_Constant1.fixedpointlog
  Constant2 : allblocks_alteradspbuilder2/Constant  mask_cst=0  BusType=Unsigned Integer  bwl=10  bwr=0  roundMode=Truncate  satMode=Wrap  SpecifyClock=off  allowFloatingPointOverride=on  logOutputs=off  logFile=C:\Users\ASUS\Desktop\sift_fpga\Octave_2\tb_test_final_sift\test%5Ffinal%5Fsift_sift%5Foctave1_matching_add%5Fread%5Fdesciptor_Constant2.fixedpointlog
  Counter : allblocks_alteradspbuilder2/Counter  BusType=Unsigned Integer  bwl=10  bwr=0  use_modulo=on  modulo=1000  SpecifyClock=off  direction=Increment  use_sload=off  use_sset=off  svalue=1  use_clk_ena=off  use_ena=on  use_sclr=on  pipeline_display=1
  Counter1 : allblocks_alteradspbuilder2/Counter  BusType=Unsigned Integer  bwl=10  bwr=0  use_modulo=on  modulo=1000  SpecifyClock=off  direction=Increment  use_sload=off  use_sset=off  svalue=0  use_clk_ena=off  use_ena=on  use_sclr=on  pipeline_display=1
  Delay : allblocks_alteradspbuilder2/Delay  pipeline=1  pipeline_display=1  ClockPhase=1  use_ena=on  use_sclr=off  allowFloatingPointOverride=on  logOutputs=off  logFile=C:\Users\ASUS\Desktop\sift_fpga\Octave_2\tb_test_final_sift\test%5Ffinal%5Fsift_sift%5Foctave1_matching_add%5Fread%5Fdesciptor_Delay.fixedpointlog  use_init=off  reset_value=1
  Logical Bit Operator{,1,3..5} (5 alike) : allblocks_alteradspbuilder2/Logical Bit Operator  LogicalOperator=AND  user_inputs=2  pipeline_display=0
  Logical Bit Operator2 : allblocks_alteradspbuilder2/Logical Bit Operator  LogicalOperator=NAND  user_inputs=2  pipeline_display=0
  Logical Bit Operator6 : allblocks_alteradspbuilder2/Logical Bit Operator  LogicalOperator=OR  user_inputs=2  pipeline_display=0
  Multiplexer : allblocks_alteradspbuilder2/Multiplexer  numInputs=2  pipeline=0  oneHot=off  pipeline_display=0  use_ena=off  use_aclr=off  allowFloatingPointOverride=on  logOutputs=off  logFile=C:\test%5Ffinal%5Fsift_sift%5Foctave1_matching_add%5Fread%5Fdesciptor_Multiplexer.fixedpointlog
  add_read_first : Outport
  add_read_second : Outport  Port=2
  rs_ram_location : Outport  Port=3
  wires:
  Logical Bit Operator/1 -> Multiplexer/3
  [add_read_first] -> Comparator/1
  option_ena/1 -> [option_ena]
  Constant/1 -> Comparator/2
  Comparator/1 -> Logical Bit Operator/2
  valid_in/1 -> [valid_in]
  Counter1/1 -> [add_read_second]
  Counter/1 -> [add_read_first]
  [add_read_second] -> add_read_second/1
  [add_read_first] -> add_read_first/1
  [reset_add_ram_location_match] -> rs_ram_location/1
  Logical Bit Operator5/1 -> Counter1/2, Counter/2
  [option_ena] -> Logical Bit Operator2/2, Logical Bit Operator2/1
  Logical Bit Operator2/1 -> Logical Bit Operator5/1
  [valid_in] -> Logical Bit Operator5/2
  [option_ena] -> Logical Bit Operator3/1
  [valid_in] -> Logical Bit Operator3/2
  Logical Bit Operator3/1 -> Delay/1
  [valid_in] -> Delay/2
  Logical Bit Operator4/1 -> Logical Bit Operator6/1
  [option_ena] -> Logical Bit Operator4/1
  [valid_in] -> Logical Bit Operator4/2
  Delay/1 -> Logical Bit Operator6/2
  Logical Bit Operator6/1 -> [ena]
  [ena] -> Counter/1, Logical Bit Operator/1
  Multiplexer/1 -> Counter1/1
  [option_ena] -> Multiplexer/1
  [ena] -> Multiplexer/2
  [add_read_first] -> Comparator1/1
  Constant1/1 -> Comparator1/2
  [add_read_second] -> Comparator2/1
  Constant2/1 -> Comparator2/2
  Comparator1/1 -> Logical Bit Operator1/1
  Comparator2/1 -> Logical Bit Operator1/2
  Logical Bit Operator1/1 -> [reset_add_ram_location_match]

== system test_final_sift/sift_octave1/matching/compare_descriptor ==
  descriptor1 : Inport
  descriptor2 : Inport  Port=2
  clken : Inport  Port=3
  threshold : Inport  Port=4
  addr1_in : Inport  Port=5
  addr2_in : Inport  Port=6
  AltBus1 : allblocks_alteradspbuilder2/AltBus  BusType=Unsigned Integer  bwl=20  bwr=0  saturate=off  floatingPointInput=on  floatingPointOutput=on  logOutputs=off  logFile=C:\Users\ASUS\Desktop\sift_fpga\Octave_2\tb_test_final_sift\test%5Ffinal%5Fsift_sift%5Foctave1_matching_compare%5Fdescriptor_AltBus1.fixedpointlog
  AltBus2 : allblocks_alteradspbuilder2/AltBus  BusType=Unsigned Integer  bwl=16  bwr=0  saturate=off  floatingPointInput=on  floatingPointOutput=on  logOutputs=off  logFile=C:\Users\ASUS\Desktop\sift_fpga\Octave_2\tb_test_final_sift\test%5Ffinal%5Fsift_sift%5Foctave1_matching_compare%5Fdescriptor_AltBus2.fixedpointlog
  AltBus3 : allblocks_alteradspbuilder2/AltBus  BusType=Unsigned Integer  bwl=16  bwr=0  saturate=off  floatingPointInput=on  floatingPointOutput=on  logOutputs=off  logFile=C:\Users\ASUS\Desktop\sift_fpga\Octave_2\tb_test_final_sift\test%5Ffinal%5Fsift_sift%5Foctave1_matching_compare%5Fdescriptor_AltBus3.fixedpointlog
  BusSplitter : Subsystem
  BusSplitter1 : Subsystem
  Delay : allblocks_alteradspbuilder2/Delay  pipeline=7  pipeline_display=7  ClockPhase=1  use_ena=on  use_sclr=off  allowFloatingPointOverride=on  logOutputs=off  logFile=C:\Users\ASUS\Desktop\sift_fpga\Octave_2\tb_test_final_sift\test%5Ffinal%5Fsift_sift%5Foctave1_matching_compare%5Fdescriptor_Delay.fixedpointlog  use_init=off  reset_value=1
  Delay1 : allblocks_alteradspbuilder2/Delay  pipeline=8  pipeline_display=8  ClockPhase=1  use_ena=on  use_sclr=off  allowFloatingPointOverride=on  logOutputs=off  logFile=C:\Users\ASUS\Desktop\sift_fpga\Octave_2\tb_test_final_sift\test%5Ffinal%5Fsift_sift%5Foctave1_matching_compare%5Fdescriptor_Delay1.fixedpointlog  use_init=off  reset_value=1
  Logical Bit Operator : allblocks_alteradspbuilder2/Logical Bit Operator  LogicalOperator=AND  user_inputs=2  pipeline_display=0
  Logical Bus Operator : allblocks_alteradspbuilder2/Logical Bus Operator  BusType=Unsigned Integer  bwl=1173  bwr=0  LogicalOp_text=AND  mask_value_num=128*9  shift_amount=3  force_sign_ext=on  pipeline_display=0
  Parallel Adder Subtractor : allblocks_alteradspbuilder2/Parallel Adder Subtractor  number_of_inputs=9  direction=+  use_pipeline=on  pipeline_display=4  phase_selection=1  use_ena=on  use_aclr=off  allowFloatingPointOverride=on  logOutputs=off  logFile=C:\Users\ASUS\Desktop\sift_fpga\Octave_2\tb_test_final_sift\test%5Ffinal%5Fsift_sift%5Foctave1_matching_compare%5Fdescriptor_Parallel+Adder+Subtractor.fixedpointlog
  compare : Subsystem
  get_distance : Subsystem
  get_distance1 : Subsystem
  get_distance2 : Subsystem
  get_distance3 : Subsystem
  get_distance4 : Subsystem
  get_distance5 : Subsystem
  get_distance6 : Subsystem
  get_distance7 : Subsystem
  get_distance8 : Subsystem
  isDescriptor : Subsystem
  match : Outport
  location : Outport  Port=2
  wires:
  descriptor1/1 -> [descriptor1]
  descriptor2/1 -> [descriptor2]
  [descriptor1] -> BusSplitter/1(descriptor_in)
  [descriptor2] -> BusSplitter1/1(descriptor_in)
  BusSplitter/1(hist1) -> [hist11]
  BusSplitter/2(hist2) -> [hist12]
  BusSplitter/3(hist3) -> [hist13]
  BusSplitter/4(hist4) -> [hist14]
  BusSplitter/5(hist5) -> [hist15]
  BusSplitter/6(hist6) -> [hist16]
  BusSplitter/7(hist7) -> [hist17]
  BusSplitter/8(hist8) -> [hist18]
  BusSplitter/9(hist9) -> [hist19]
  BusSplitter1/1(hist1) -> [hist21]
  BusSplitter1/2(hist2) -> [hist22]
  BusSplitter1/3(hist3) -> [hist23]
  BusSplitter1/4(hist4) -> [hist24]
  BusSplitter1/5(hist5) -> [hist25]
  BusSplitter1/6(hist6) -> [hist26]
  BusSplitter1/7(hist7) -> [hist27]
  BusSplitter1/8(hist8) -> [hist28]
  BusSplitter1/9(hist9) -> [hist29]
  clken/1 -> [clken]
  [clken] -> get_distance/3(clken)
  [hist21] -> get_distance/2(hist_in2)
  [hist11] -> get_distance/1(hist_in1)
  get_distance/1(distance_out) -> [distance1]
  [clken] -> get_distance1/3(clken)
  [hist22] -> get_distance1/2(hist_in2)
  [hist12] -> get_distance1/1(hist_in1)
  get_distance1/1(distance_out) -> [distance2]
  [clken] -> get_distance2/3(clken)
  [hist23] -> get_distance2/2(hist_in2)
  [hist13] -> get_distance2/1(hist_in1)
  get_distance2/1(distance_out) -> [distance3]
  [clken] -> get_distance3/3(clken)
  [hist24] -> get_distance3/2(hist_in2)
  [hist14] -> get_distance3/1(hist_in1)
  get_distance3/1(distance_out) -> [distance4]
  [clken] -> get_distance4/3(clken)
  [hist25] -> get_distance4/2(hist_in2)
  [hist15] -> get_distance4/1(hist_in1)
  get_distance4/1(distance_out) -> [distance5]
  [clken] -> get_distance5/3(clken)
  [hist26] -> get_distance5/2(hist_in2)
  [hist16] -> get_distance5/1(hist_in1)
  get_distance5/1(distance_out) -> [distance6]
  [clken] -> get_distance6/3(clken)
  [hist27] -> get_distance6/2(hist_in2)
  [hist17] -> get_distance6/1(hist_in1)
  get_distance6/1(distance_out) -> [distance7]
  [clken] -> get_distance7/3(clken)
  [hist28] -> get_distance7/2(hist_in2)
  [hist18] -> get_distance7/1(hist_in1)
  get_distance7/1(distance_out) -> [distance8]
  [clken] -> get_distance8/3(clken)
  [hist29] -> get_distance8/2(hist_in2)
  [hist19] -> get_distance8/1(hist_in1)
  get_distance8/1(distance_out) -> [distance9]
  [distance1] -> Parallel Adder Subtractor/1
  [distance2] -> Parallel Adder Subtractor/2
  [distance3] -> Parallel Adder Subtractor/3
  [distance4] -> Parallel Adder Subtractor/4
  [distance5] -> Parallel Adder Subtractor/5
  [distance6] -> Parallel Adder Subtractor/6
  [distance7] -> Parallel Adder Subtractor/7
  [distance8] -> Parallel Adder Subtractor/8
  [distance9] -> Parallel Adder Subtractor/9
  [clken] -> Parallel Adder Subtractor/10
  threshold/1 -> [threshold]
  [distance] -> AltBus3/1
  [threshold] -> AltBus2/1
  compare/1(match) -> Logical Bit Operator/2
  [descriptor2] -> Delay1/1
  Logical Bus Operator/1 -> AltBus1/1
  AltBus1/1 -> [location]
  [location] -> location/1
  [match] -> match/1
  addr1_in/1 -> [addr1_in]
  addr2_in/1 -> [addr2_in]
  [descriptor1] -> isDescriptor/1(descriptor1)
  [descriptor2] -> isDescriptor/2(descriptor2)
  [addr1_in] -> isDescriptor/3(addr1_in)
  [addr2_in] -> isDescriptor/4(addr2_in)
  isDescriptor/1(isDescriptor) -> Delay/1
  Logical Bit Operator/1 -> [match]
  Delay/1 -> Logical Bit Operator/1
  [clken] -> Delay/2
  Delay1/1 -> Logical Bus Operator/1
  [clken] -> Delay1/2
  Parallel Adder Subtractor/1 -> [distance]
  AltBus2/1 -> compare/1(threshold)
  AltBus3/1 -> compare/2(distance)
